simulink model "succ_loop_sim"  (R2019b)
settings: Solver=VariableStepAuto  StartTime=0.0  StopTime=100  RelTol=1e-3
values from neighbouring files (symbols this model uses):
  a1 = 2.87    [oppg2c.m]    (also in oppg2e.m; oppg2f.m)
  a2 = -0.65    [oppg2c.m]    (also in oppg2e.m; oppg2f.m)
  dist = 1.5    [oppg2e.m]    (also in oppg2f.m)
  g = 9.81    [oppg2e.m]    (also in oppg2f.m)
  Kd_phi = 1.935    [oppg2e.m]    (also in oppg2f.m)
  Ki_phi = 0    [oppg2e.m]    (also in oppg2f.m)
  Ki_x = omega_n_x^2 *Vg/g    (= 0.213420550459)    [oppg2e.m]    (also in oppg2f.m)
  Kp_phi = -2    [oppg2e.m]    (also in oppg2f.m)
  Kp_x = 2*zeta_x*omega_n_x*Vg/g    (= 7.48844036697)    [oppg2e.m]    (also in oppg2f.m)
  Vg = 161.1    [oppg2e.m]    (also in oppg2f.m)
settings Model: Creator=jacob  LastModifiedBy=jacob

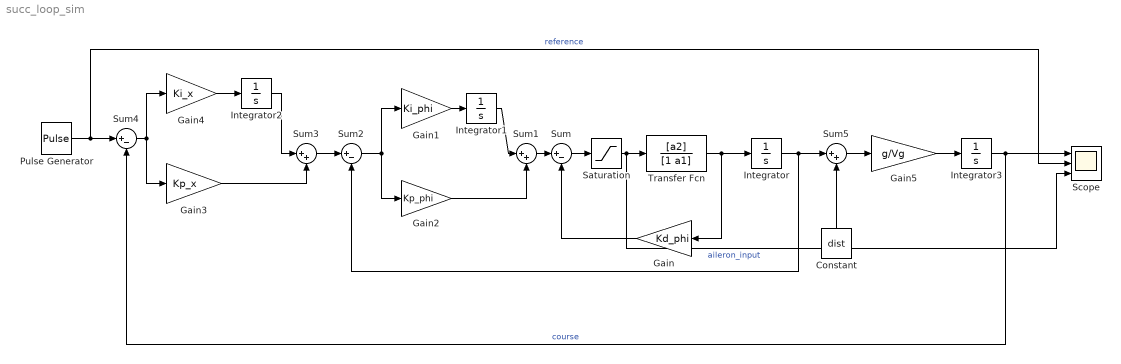
== system succ_loop_sim ==
  Constant : Constant  Value=dist
  Gain : Gain  Gain=Kd_phi
  Gain1 : Gain  Gain=Ki_phi
  Gain2 : Gain  Gain=Kp_phi
  Gain3 : Gain  Gain=Kp_x
  Gain4 : Gain  Gain=Ki_x
  Gain5 : Gain  Gain=g/Vg
  Integrator{,1..3} (4 alike) : Integrator
  Pulse Generator : DiscretePulseGenerator  PulseType=Time based  Amplitude=10  Period=50  PulseWidth=50
  Saturation : Saturate  UpperLimit=30  LowerLimit=-30
  Scope : Scope  NumInputPorts=3
  Sum : Sum  Inputs=|+-
  Sum1 : Sum  Inputs=|++
  Sum2 : Sum  Inputs=|+-
  Sum3 : Sum  Inputs=|++
  Sum4 : Sum  Inputs=|+-
  Sum5 : Sum  Inputs=|++
  Transfer Fcn : TransferFcn  Numerator=[a2]  Denominator=[1 a1]
  wires:
  Transfer Fcn/1 -> Integrator/1, Gain/1
  Gain/1 -> Sum/2
  Gain1/1 -> Integrator1/1
  Sum1/1 -> Sum/1
  Integrator1/1 -> Sum1/1
  Gain2/1 -> Sum1/2
  Integrator/1 -> Sum2/2, Sum5/1
  Sum3/1 -> Sum2/1
  Gain3/1 -> Sum3/2
  Gain4/1 -> Integrator2/1
  Integrator2/1 -> Sum3/1
  Constant/1 -> Sum5/2
  Sum5/1 -> Gain5/1
  Gain5/1 -> Integrator3/1
  Integrator3/1 -> Sum4/2, Scope/1  "course"
  Pulse Generator/1 -> Scope/2, Sum4/1  "reference"
  Sum/1 -> Saturation/1
  Saturation/1 -> Scope/3, Transfer Fcn/1  "aileron_input"
  Sum4/1 -> Gain3/1, Gain4/1
  Sum2/1 -> Gain2/1, Gain1/1
